simulink model "rtwdemo_slexprfold"  (Simulink 7.6)
settings: Solver=FixedStepDiscrete  StartTime=0.0  StopTime=10.0  RelTol=1e-3  SampleTimeConstraint=STIndependent
PreLoadFcn:
  | rtwdemo_slexprfold_data
undefined symbols (not defined in the file or in its folder): LOWER, T1Break, T1Data, T2Data, UPPER
libraries: rtwdemowidgets x2
Description:
  | Expression Folding in Generated Code
settings Model: Creator=The MathWorks Inc.  CovMetricSettings=d  ExtModeAutoUpdateStatusClock=off
settings DataIOCC: SaveOutput=off  SaveTime=off  SignalLoggingName=sigsOut
settings OptimizationCC: InlineParams=on  InlineInvariantSignals=on  StateBitsets=on  DataBitsets=on  UseTempVars=on  EfficientFloat2IntCast=on  EfficientMapNaN2IntZero=off
settings DebuggingCC: CheckExecutionContextPreStartOutputMsg=on  CheckExecutionContextRuntimeOutputMsg=on  SolverPrmCheckMsg=none  StrictBusMsg=ErrorOnBusTreatedAsVector
settings HardwareCC: ProdIntDivRoundTo=Zero  ProdEndianess=LittleEndian  ProdHWDeviceType=Generic->32-bit Embedded Processor  TargetHWDeviceType=Generic->32-bit Embedded Processor
settings RTWCC: TLCOptions=-p0 -aWarnNonSaturatedBlocks=0  GenerateReport=on  RTWVerbose=off  ProcessScript=grt_make_rtw_hook  LaunchReport=on
settings CodeAppCC: ForceParamTrailComments=on
settings GRTTargetCC: TargetFcnLib=ansi_tfl_tmw.mat

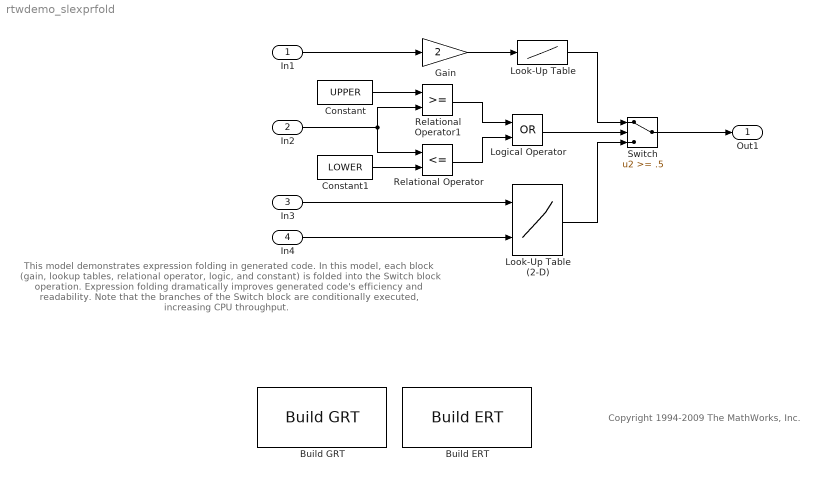
== system rtwdemo_slexprfold ==
  note: This model demonstrates expression folding in generated code.  In this model, each
      | block (gain, lookup tables, relational operator, logic, and constant) is folded into the
      | Switch block operation.  Expression folding dramatically improves generated code's
      | efficiency and readability.  Note that the branches of the Switch block are conditionally
      | executed, increasing CPU throughput.
  note: Copyright 1994-2009 The MathWorks, Inc.
  In1 : Inport  OutDataTypeStr=double  PortDimensions=1
  In2 : Inport  Port=2  OutDataTypeStr=double  PortDimensions=1
  In3 : Inport  Port=3  OutDataTypeStr=double  PortDimensions=1
  In4 : Inport  Port=4  OutDataTypeStr=double  PortDimensions=1
  Build ERT : rtwdemowidgets/Build ERT  SystemSampleTime=-1  attrib_overrides={}
  Build GRT : rtwdemowidgets/Build GRT  SystemSampleTime=-1  attrib_overrides={}
  Constant : Constant  Value=UPPER
  Constant1 : Constant  Value=LOWER
  Gain : Gain  Gain=2  SaturateOnIntegerOverflow=on  OutDataTypeStr=Inherit: Same as input  ParamDataTypeStr=Inherit: Same as input
  Logical Operator : Logic  Operator=OR
  Look-Up Table : Lookup  InputValues=T1Break  Table=T1Data  SaturateOnIntegerOverflow=on
  Look-Up Table (2-D) : Lookup2D  RowIndex=T2Break  ColumnIndex=T2Break  Table=T2Data  InputSameDT=on
  Relational Operator : RelationalOperator  Operator=<=  InputSameDT=on
  Relational Operator1 : RelationalOperator  InputSameDT=on
  Switch : Switch  Threshold=.5  SaturateOnIntegerOverflow=on  InputSameDT=on
  Out1 : Outport
  wires:
  Relational Operator1/1 -> Logical Operator/1
  Relational Operator/1 -> Logical Operator/2
  Logical Operator/1 -> Switch/2
  Constant1/1 -> Relational Operator/2
  In1/1 -> Gain/1
  Look-Up Table/1 -> Switch/1
  Switch/1 -> Out1/1
  Gain/1 -> Look-Up Table/1
  Look-Up Table (2-D)/1 -> Switch/3
  Constant/1 -> Relational Operator1/1
  In2/1 -> Relational Operator1/2, Relational Operator/1
  In3/1 -> Look-Up Table (2-D)/1
  In4/1 -> Look-Up Table (2-D)/2
